simulink model "Ex_Jun_2023_2"  (R2022b)
settings: Solver=VariableStepAuto  StartTime=0.0  StopTime=150  RelTol=1e-3
settings Model: Creator=rrilo  LastModifiedBy=rrilo

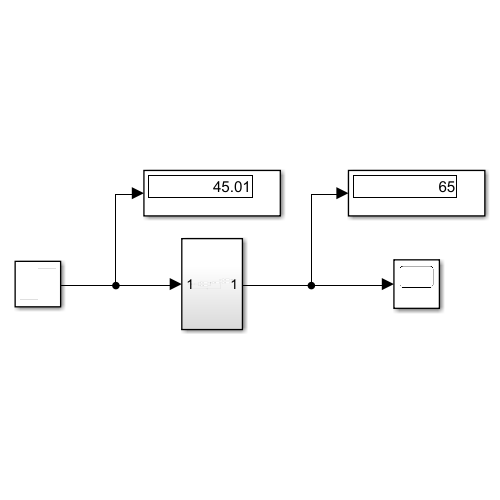
[thumbnail: Simulink's stored preview of the top-level diagram]
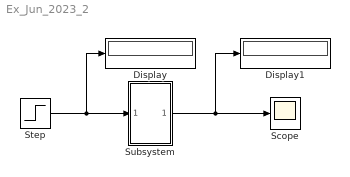
== system Ex_Jun_2023_2 ==
  Display : Display
  Display1 : Display
  Scope : Scope
  Step : Step  After=45.008  SampleTime=0
  Subsystem : Subsystem
  wires:
  Subsystem/1(Out1) -> Display1/1, Scope/1
  Step/1 -> Display/1, Subsystem/1(In1)

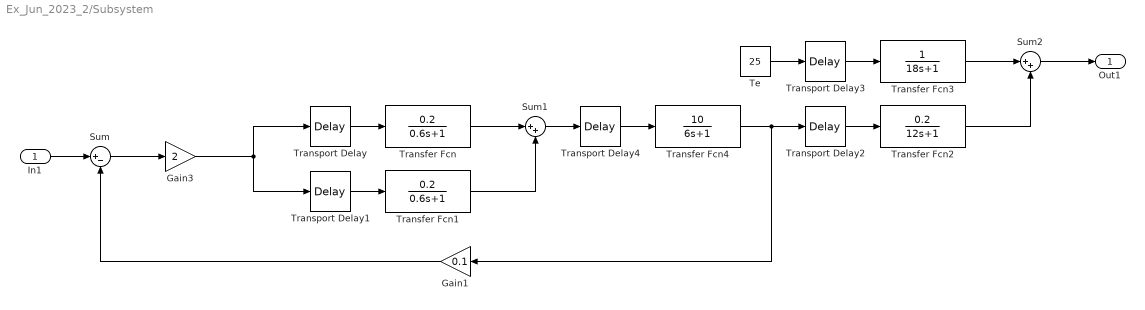
== system Ex_Jun_2023_2/Subsystem ==
  In1 : Inport
  Gain1 : Gain  Gain=0.1
  Gain3 : Gain  Gain=2
  Sum : Sum  Inputs=|+-
  Sum1 : Sum  Inputs=|++
  Sum2 : Sum  Inputs=|++
  Te : Constant  Value=25
  Transfer Fcn : TransferFcn  Numerator=[0.2]  Denominator=[0.6 1]
  Transfer Fcn1 : TransferFcn  Numerator=[0.2]  Denominator=[0.6 1]
  Transfer Fcn2 : TransferFcn  Numerator=[0.2]  Denominator=[12 1]
  Transfer Fcn3 : TransferFcn  Denominator=[18 1]
  Transfer Fcn4 : TransferFcn  Numerator=[10]  Denominator=[6 1]
  Transport Delay : TransportDelay  DelayTime=0.2
  Transport Delay1 : TransportDelay  DelayTime=0.5
  Transport Delay2 : TransportDelay
  Transport Delay3 : TransportDelay  DelayTime=5.5
  Transport Delay4 : TransportDelay
  Out1 : Outport
  wires:
  Sum2/1 -> Out1/1
  Transport Delay/1 -> Transfer Fcn/1
  Transport Delay1/1 -> Transfer Fcn1/1
  Transport Delay2/1 -> Transfer Fcn2/1
  Transport Delay3/1 -> Transfer Fcn3/1
  Transport Delay4/1 -> Transfer Fcn4/1
  In1/1 -> Sum/1
  Gain1/1 -> Sum/2
  Sum/1 -> Gain3/1
  Gain3/1 -> Transport Delay1/1, Transport Delay/1
  Transfer Fcn/1 -> Sum1/1
  Transfer Fcn1/1 -> Sum1/2
  Sum1/1 -> Transport Delay4/1
  Transfer Fcn4/1 -> Gain1/1, Transport Delay2/1
  Transfer Fcn3/1 -> Sum2/1
  Transfer Fcn2/1 -> Sum2/2
  Te/1 -> Transport Delay3/1
